simulink model "rst_modular_test"  (R2023b)
settings: Solver=VariableStepAuto  StartTime=0.0  StopTime=tt1+2*tt1+2*tt2+2*100 + tt2/2  RelTol=1e-3
values from neighbouring files (symbols this model uses):
  A = A(1:na+1)    [rst.m]    (also in rst_int.m = A* Hs; script2_waterloo.m = m_bj.F; untitled.m)
  Am = H01.Denominator{1}    [untitled.m]
  amp2 = amp/dcgain(m_final)    [script.m]    (also in script2_waterloo.m = amp/dcgain(m_bj))
  B = m_bj.B * amp2    [script2_waterloo.m]
  Bm = H01.Numerator{1}    [untitled.m]
  r = 173    [script2_waterloo.m]    (also in untitled.m = 50)
  T = t(2)-t(1)    [frecventa.m]    (also in rst.m = sum(P)/sum(B); rst_int.m = sum(P)/sum(B); untitled.m = sum(P)/sum(B))
  Te = 5    [Ursu_spab_60min.mat]    (also in script.m; script2_waterloo.m = m_bj.Ts; test_merge.mat = 1; untitled.m = 0.1)
  tt1 = 33    [script2_waterloo.m]    (also in untitled.m = 11)
  tt2 = 330    [script2_waterloo.m]    (also in untitled.m = 6)
  y_st = 15.62    [script.m]    (also in script2_waterloo.m = 15.2)
undefined symbols (not defined in the file or in its folder): m_bj
settings Model: Creator=wombelbat  LastModifiedBy=wombelbat

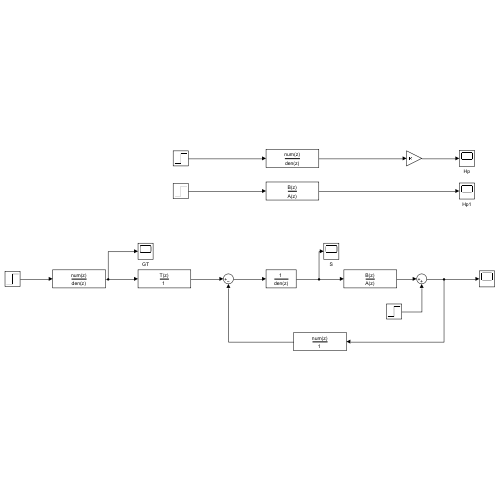
[thumbnail: Simulink's stored preview of the top-level diagram]
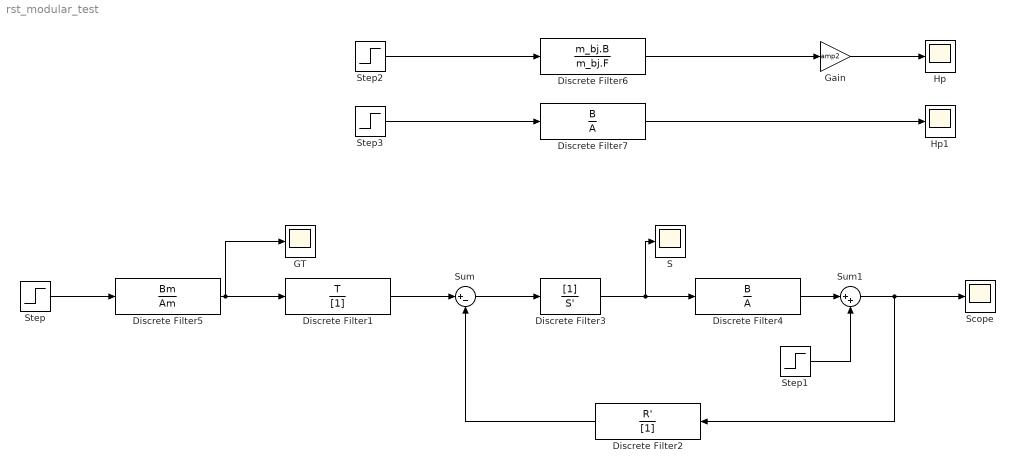
== system rst_modular_test ==
  Discrete Filter1 : DiscreteFilter  Numerator=T  Denominator=[1]
  Discrete Filter2 : DiscreteFilter  Numerator=R'  Denominator=[1]
  Discrete Filter3 : DiscreteFilter  Denominator=S'
  Discrete Filter4 : DiscreteFilter  Numerator=B  Denominator=A
  Discrete Filter5 : DiscreteFilter  Numerator=Bm  Denominator=Am
  Discrete Filter6 : DiscreteFilter  Numerator=m_bj.B  Denominator=m_bj.F
  Discrete Filter7 : DiscreteFilter  Numerator=B  Denominator=A
  GT : Scope
  Gain : Gain  Gain=amp2
  Hp : Scope
  Hp1 : Scope
  S : Scope
  Scope : Scope
  Step : Step  Time=0  After=y_st  SampleTime=Te
  Step1 : Step  Time=tt1+tt2+tt2+100  After=0.2*r  SampleTime=Te
  Step2 : Step  Time=0  After=173  SampleTime=Te
  Step3 : Step  Time=0  After=173  SampleTime=Te
  Sum : Sum  Inputs=|+-
  Sum1 : Sum  Inputs=|++
  wires:
  Step/1 -> Discrete Filter5/1
  Discrete Filter3/1 -> S/1, Discrete Filter4/1
  Sum/1 -> Discrete Filter3/1
  Discrete Filter1/1 -> Sum/1
  Discrete Filter2/1 -> Sum/2
  Discrete Filter4/1 -> Sum1/1
  Step1/1 -> Sum1/2
  Sum1/1 -> Discrete Filter2/1, Scope/1
  Step2/1 -> Discrete Filter6/1
  Discrete Filter5/1 -> GT/1, Discrete Filter1/1
  Discrete Filter6/1 -> Gain/1
  Gain/1 -> Hp/1
  Step3/1 -> Discrete Filter7/1
  Discrete Filter7/1 -> Hp1/1
